simulink model "Simulador_No_lineal"  (R2023a)
settings: Solver=FixedStepAuto  StartTime=0.0  StopTime=70  FixedStep=Ts  RelTol=1e-3
undefined symbols (not defined in the file): IMU1_aB, IMU1_aK, IMU1_aN, IMU1_gB, IMU1_gK, IMU1_gN, IMU2_aB, IMU2_aK, IMU2_aN, IMU2_gB, IMU2_gK, IMU2_gN, IMU3_aB, IMU3_aK, IMU3_aN, IMU3_gB, IMU3_gK, IMU3_gN, Ts, TsMot, TsPos, TsRef, TsSenB, TsSenF, TsVel
libraries: mspsensorlib x3, simulink x1
(part 1 of 3)
settings Model: Creator=rrico  LastModifiedBy=rrico
settings OptimizationCC: ReuseModelBlockBuffer=off

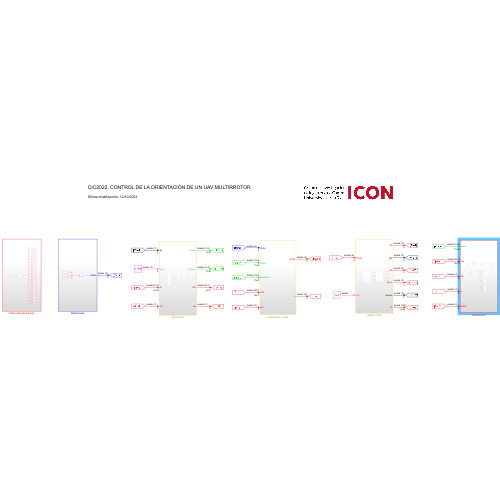
[thumbnail: Simulink's stored preview of the top-level diagram]
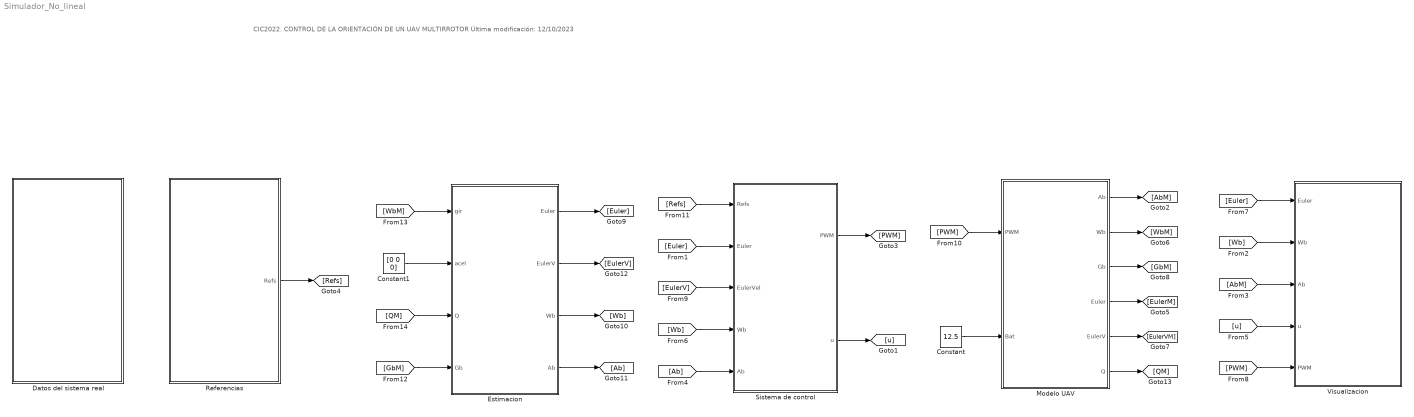
== system Simulador_No_lineal ==
  note: CIC2022. CONTROL DE LA ORIENTACIÓN DE UN UAV MULTIRROTOR
      |
      | Última modificación: 12/10/2023
  Constant : Constant  Value=12.5
  Constant1 : Constant  Value=[0 0 0]
  Datos del sistema real : Subsystem
  Estimacion : Subsystem
  Modelo UAV : Subsystem
  Referencias : Subsystem
  Sistema de control : Subsystem
  Visualizacion : Subsystem
  wires:
  Referencias/1(Refs) -> [Refs]
  [Wb] -> Visualizacion/2(Wb)
  [AbM] -> Visualizacion/3(Ab)
  [PWM] -> Visualizacion/5(PWM)
  [u] -> Visualizacion/4(u)
  Constant/1 -> Modelo UAV/2(Bat)
  Sistema de control/1(PWM) -> [PWM]
  [PWM] -> Modelo UAV/1(PWM)
  Modelo UAV/2(Wb) -> [WbM]
  Modelo UAV/1(Ab) -> [AbM]
  [Refs] -> Sistema de control/1(Refs)
  [Wb] -> Sistema de control/4(Wb)
  Sistema de control/2(u) -> [u]
  [Euler] -> Sistema de control/2(Euler)
  Modelo UAV/4(Euler) -> [EulerM]
  [Euler] -> Visualizacion/1(Euler)
  [Ab] -> Sistema de control/5(Ab)
  Modelo UAV/5(EulerV) -> [EulerVM]
  [EulerV] -> Sistema de control/3(EulerVel)
  Modelo UAV/3(Gb) -> [GbM]
  [WbM] -> Estimacion/1(gir)
  Constant1/1 -> Estimacion/2(acel)
  Estimacion/1(Euler) -> [Euler]
  Estimacion/3(Wb) -> [Wb]
  Estimacion/4(Ab) -> [Ab]
  Estimacion/2(EulerV) -> [EulerV]
  Modelo UAV/6(Q) -> [QM]
  [QM] -> Estimacion/3(Q)
  [GbM] -> Estimacion/4(Gb)

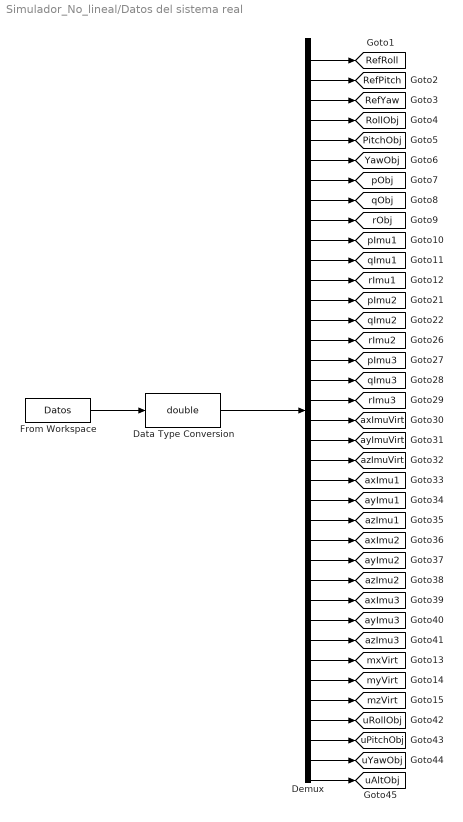
== system Simulador_No_lineal/Datos del sistema real ==
  Data Type Conversion : DataTypeConversion  OutDataTypeStr=double  SaturateOnIntegerOverflow=off  RndMeth=Floor
  Demux : Demux  Outputs=38
  From Workspace : FromWorkspace  VariableName=Datos  SampleTime=Ts
  tag scope: PitchObj=global, RefPitch=global, RefRoll=global, RefYaw=global, RollObj=global, YawObj=global, axImu1=global, axImu2=global, axImu3=global, axImuVirt=global, ayImu1=global, ayImu2=global, ayImu3=global, ayImuVirt=global, azImu1=global, azImu2=global, azImu3=global, azImuVirt=global, mxVirt=global, myVirt=global, mzVirt=global, pImu1=global, pImu2=global, pImu3=global, pObj=global, qImu1=global, qImu2=global, qImu3=global, qObj=global, rImu1=global, rImu2=global, rImu3=global, rObj=global, uAltObj=global, uPitchObj=global, uRollObj=global, uYawObj=global
  wires:
  Demux/31 -> [azImu3]
  Demux/7 -> [YawObj]
  Demux/17 -> [pImu3]
  Demux/25 -> [azImu1]
  Demux/27 -> [ayImu2]
  Demux/16 -> [rImu2]
  Demux/15 -> [qImu2]
  Demux/30 -> [ayImu3]
  Demux/21 -> [ayImuVirt]
  Demux/10 -> [rObj]
  Demux/2 -> [RefRoll]
  Demux/24 -> [ayImu1]
  Demux/5 -> [RollObj]
  Demux/29 -> [axImu3]
  Demux/8 -> [pObj]
  Demux/28 -> [azImu2]
  Demux/18 -> [qImu3]
  Demux/6 -> [PitchObj]
  Demux/19 -> [rImu3]
  Data Type Conversion/1 -> Demux/1
  Demux/4 -> [RefYaw]
  Demux/22 -> [azImuVirt]
  From Workspace/1 -> Data Type Conversion/1
  Demux/23 -> [axImu1]
  Demux/9 -> [qObj]
  Demux/13 -> [rImu1]
  Demux/3 -> [RefPitch]
  Demux/26 -> [axImu2]
  Demux/11 -> [pImu1]
  Demux/14 -> [pImu2]
  Demux/38 -> [uAltObj]
  Demux/37 -> [uYawObj]
  Demux/36 -> [uPitchObj]
  Demux/35 -> [uRollObj]
  Demux/32 -> [mxVirt]
  Demux/33 -> [myVirt]
  Demux/34 -> [mzVirt]
  Demux/20 -> [axImuVirt]
  Demux/12 -> [qImu1]

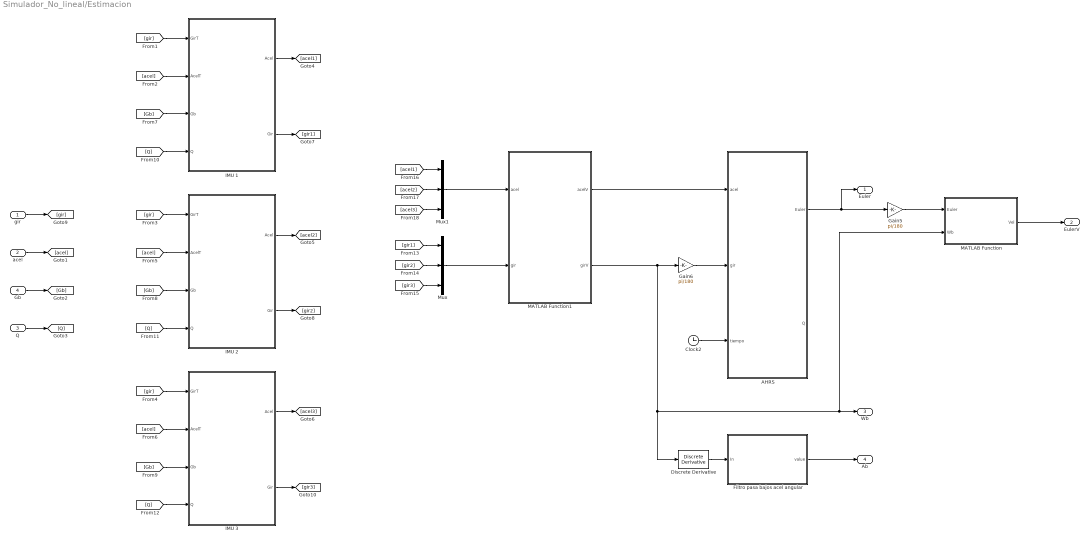
== system Simulador_No_lineal/Estimacion ==
  gir : Inport
  acel : Inport  Port=2
  Q : Inport  Port=3
  Gb : Inport  Port=4
  AHRS : Subsystem  TreatAsAtomicUnit=on  SystemSampleTime=TsPos  mask{T=on, Beta=0.033, Zeta=0.005, Kp=0.5, Ki=0.1}
      mask prompts: T "Filtro Madgwick"
  Clock2 : Clock
  Discrete Derivative : simulink/Discrete/Discrete Derivative  gainval=1.0  ICPrevScaledInput=0.0  OutMin=[]  OutMax=[]  OutDataType=fixdt(1, 16)  OutScaling=2^-10  DoSatur=off
  Filtro pasa bajos acel angular : Subsystem  TreatAsAtomicUnit=on  SystemSampleTime=TsVel  mask{P=2, Fc=30, TsF=TsSenF}
      mask prompts: P "Polos"; Fc "Frecuencia de corte"; TsF "Tiempo de muestreo"
      mask DialogControl ParameterGroup1 Prompt: Parameters
  Gain5 : Gain  Gain=pi/180
  Gain6 : Gain  Gain=pi/180
  IMU 1 : Subsystem  mask{aN=IMU1_aN, aB=IMU1_aB, aK=IMU1_aK, gN=IMU1_gN, gB=IMU1_gB, gK=IMU1_gK, E=on, R=off, ESM=on, EF=on, NP=2, FC=40}
      mask prompts: aN "Velocity random walk"; aB "Bias instability"; aK "Acceleration random walk"; gN "Angle random walk"; gB "Bias instability"; gK "Rate random walk"; E "Activar IMU"; R "Activar ruido externo"; ESM "Activar submuestreo"; EF "Activar filtro"; NP "Numero de polos"; FC "Frecuencia de corte"
      mask DialogControl ParameterGroupVar Prompt: Acelerometro
      mask DialogControl Container3 Prompt: Giroscopio
      mask DialogControl Container4 Prompt: IMU
      mask DialogControl Container5 Prompt: Filtro
  IMU 2 : Subsystem  mask{aN=IMU2_aN, aB=IMU2_aB, aK=IMU2_aK, gN=IMU2_gN, gB=IMU2_gB, gK=IMU2_gK, E=on, R=off, ESM=on, EF=on, NP=2, FC=40}
      mask prompts: aN "Velocity random walk"; aB "Bias instability"; aK "Acceleration random walk"; gN "Angle random walk"; gB "Bias instability"; gK "Rate random walk"; E "Activar IMU"; R "Activar ruido externo"; ESM "Activar submuestreo"; EF "Activar filtro"; NP "Numero de polos"; FC "Frecuencia de corte"
      mask DialogControl ParameterGroupVar Prompt: Acelerometro
      mask DialogControl Container3 Prompt: Giroscopio
      mask DialogControl Container4 Prompt: IMU
      mask DialogControl Container5 Prompt: Filtro
  IMU 3 : Subsystem  mask{aN=IMU3_aN, aB=IMU3_aB, aK=IMU3_aK, gN=IMU3_gN, gB=IMU3_gB, gK=IMU3_gK, E=on, R=off, ESM=on, EF=on, NP=2, FC=40}
      mask prompts: aN "Velocity random walk"; aB "Bias instability"; aK "Acceleration random walk"; gN "Angle random walk"; gB "Bias instability"; gK "Rate random walk"; E "Activar IMU"; R "Activar ruido externo"; ESM "Activar submuestreo"; EF "Activar filtro"; NP "Numero de polos"; FC "Frecuencia de corte"
      mask DialogControl ParameterGroupVar Prompt: Acelerometro
      mask DialogControl Container3 Prompt: Giroscopio
      mask DialogControl Container4 Prompt: IMU
      mask DialogControl Container5 Prompt: Filtro
  MATLAB Function : MATLAB Function  TreatAsAtomicUnit=on  SystemSampleTime=TsPos
  MATLAB Function1 : MATLAB Function  TreatAsAtomicUnit=on  SystemSampleTime=TsSenF
  Mux : Mux  Inputs=3
  Mux1 : Mux  Inputs=3
  Euler : Outport
  EulerV : Outport  Port=2
  Wb : Outport  Port=3
  Ab : Outport  Port=4
  wires:
  Gain6/1 -> AHRS/2(gir)
  AHRS/1(Euler) -> Euler/1, Gain5/1
  Gain5/1 -> MATLAB Function/1(Euler)
  MATLAB Function/1(Vel) -> EulerV/1
  Discrete Derivative/1 -> Filtro pasa bajos acel angular/1(In)
  Filtro pasa bajos acel angular/1(value) -> Ab/1
  Clock2/1 -> AHRS/3(tiempo)
  MATLAB Function1/2(girV) -> Wb/1, MATLAB Function/2(Wb), Discrete Derivative/1, Gain6/1
  gir/1 -> [gir]
  acel/1 -> [acel]
  Gb/1 -> [Gb]
  Q/1 -> [Q]
  [gir] -> IMU 1/1(GirT)
  [gir] -> IMU 2/1(GirT)
  [gir] -> IMU 3/1(GirT)
  [acel] -> IMU 1/2(AcelT)
  [acel] -> IMU 2/2(AcelT)
  [acel] -> IMU 3/2(AcelT)
  [Gb] -> IMU 1/3(Gb)
  [Gb] -> IMU 2/3(Gb)
  [Gb] -> IMU 3/3(Gb)
  [Q] -> IMU 1/4(Q)
  [Q] -> IMU 2/4(Q)
  [Q] -> IMU 3/4(Q)
  IMU 1/1(Acel) -> [acel1]
  IMU 2/1(Acel) -> [acel2]
  IMU 3/1(Acel) -> [acel3]
  IMU 1/2(Gir) -> [gir1]
  IMU 2/2(Gir) -> [gir2]
  IMU 3/2(Gir) -> [gir3]
  [gir1] -> Mux/1
  [gir2] -> Mux/2
  [gir3] -> Mux/3
  [acel1] -> Mux1/1
  [acel2] -> Mux1/2
  [acel3] -> Mux1/3
  Mux1/1 -> MATLAB Function1/1(acel)
  Mux/1 -> MATLAB Function1/2(gir)
  MATLAB Function1/1(acelV) -> AHRS/1(acel)

== system Simulador_No_lineal/Modelo UAV ==
  PWM : Inport
  Bat : Inport  Port=2
  Dinamica UAV : Subsystem  mask{Mo=[0 0 0], B=[0.002 0.005 0.005]*0, F=[0.025 0.006 0.006]*0, I=[0.0014 0.025 0.0549], Im=0.0005, dM=0, M=0.2472, Dr=0.09, Dp=0.0675, Y=off, Mq=on}
      mask prompts: Mo "Par inicial"; B "Rozamiento viscoso"; F "Rozamiento estático"; I "Inercia"; Im "Inercia del rotor"; dM "Distancia del centro de masas"; M "Masa"; Dr "Distancia de los rotores a roll"; Dp "Distancia de los rotores a pitch"; Y "Habilitacion yaw"; Mq "Modelo de maqueta"
      mask DialogControl DescTextVar Prompt: Modelo dinámico del UAV
      mask DialogControl Parameter1 Prompt: Rozamientos y pares adicionales
      mask DialogControl Parameter2 Prompt: Parámetros físicos
      mask DialogControl Parameter3 Prompt: Selectores
  Sistema de propulsion : Subsystem  mask{MF=[-6.7899 14.607 -0.4253 0.0213; -8.4461 16.962 -0.2084 0.0076; -9.5828 18.733 0.1539 -0.0175; -12.165 22.368 -0.0708 -0.018; -12.638 23.102 0.6345 -0.0512], MD=[0.0103 0.0273 0.0082 0.0004; -0.0179 0.0606 0.005 0.0001; 0.0107 0.032 0.0095 0.0002; -0.0117 0.0697 0.0007 0.0007; 0.0227 0.0301 0.0117 -0.0002], MV=[0 -1075.7 3391.3 5.1514; 0 -1117.8 3467.7 31.49; 0 -1464 4031.2 0.4344; 0 -1601.8 4277.8 4.6327; 0 -1710.5 4430.8 10.996], Vmin=12.5, Vmax=16.5, Tau=0.05}
      mask prompts: MF "Matriz de coeficientes fuerza"; MD "Matriz de coeficientes drag"; MV "Matriz de coeficientes velocidad"; Vmin "Voltaje minimo"; Vmax "Voltaje maximo"; Tau "Dinamica"
      mask DialogControl ParameterGroupVar1 Prompt: Estatica del motor
      mask DialogControl ParameterGroupVar2 Prompt: Dinamica del motor
  Ab : Outport
  Wb : Outport  Port=2
  Gb : Outport  Port=3
  Euler : Outport  Port=4
  EulerV : Outport  Port=5
  Q : Outport  Port=6
  wires:
  PWM/1 -> Sistema de propulsion/1(PWM)
  Bat/1 -> Sistema de propulsion/2(v)
  Dinamica UAV/3(Gb) -> Gb/1
  Sistema de propulsion/2(D) -> Dinamica UAV/2(Delta)
  Sistema de propulsion/3(W) -> Dinamica UAV/3(Wm)
  Dinamica UAV/2(Wb) -> Wb/1
  Sistema de propulsion/1(T) -> Dinamica UAV/1(T)
  Dinamica UAV/1(Ab) -> Ab/1
  Dinamica UAV/4(Euler) -> Euler/1
  Dinamica UAV/5(EulerV) -> EulerV/1
  Dinamica UAV/6(Q) -> Q/1

== system Simulador_No_lineal/Referencias ==
  Mux17 : Mux  Inputs=3
  Zero-Order Hold : ZeroOrderHold  SampleTime=TsRef
  Refs : Outport  VectorParamsAs1DForOutWhenUnconnected=off
  wires:
  Zero-Order Hold/1 -> Refs/1
  [RefYaw] -> Mux17/3
  [RefPitch] -> Mux17/2
  [RefRoll] -> Mux17/1
  Mux17/1 -> Zero-Order Hold/1

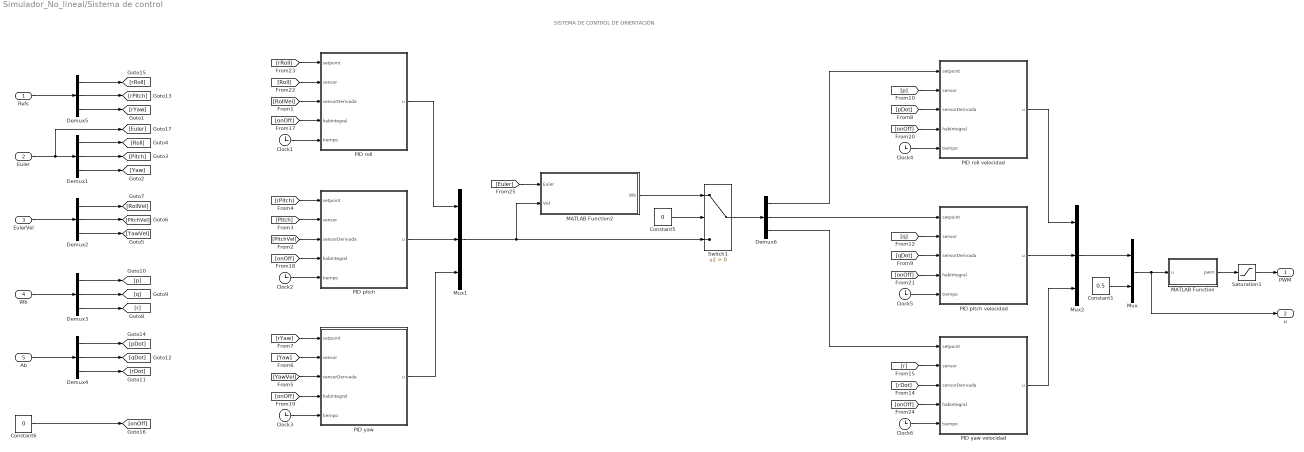
== system Simulador_No_lineal/Sistema de control ==
  note: SISTEMA DE CONTROL DE ORIENTACIÓN
  Refs : Inport
  Euler : Inport  Port=2
  EulerVel : Inport  Port=3
  Wb : Inport  Port=4
  Ab : Inport  Port=5
  Clock{1..6} (6 alike) : Clock
  Constant1 : Constant  Value=0.5  SampleTime=-1
  Constant5 : Constant  Value=0
  Constant6 : Constant  Value=0  SampleTime=-1
  Demux{1..6} (6 alike) : Demux  Outputs=3
  MATLAB Function : MATLAB Function  TreatAsAtomicUnit=on
  MATLAB Function2 : MATLAB Function  TreatAsAtomicUnit=on  SystemSampleTime=TsVel
  Mux : Mux  Inputs=2
  Mux1 : Mux  Inputs=3
  Mux2 : Mux  Inputs=3
  PID pitch : Subsystem  TreatAsAtomicUnit=on  SystemSampleTime=TsPos  mask{Kp=4, Ki=0, Kd=0, Kff=0, LimI=2000, LimT=2000}
      mask prompts: LimI "Limite I"; LimT "Limite total"
  PID pitch velocidad : Subsystem  TreatAsAtomicUnit=on  SystemSampleTime=TsVel  mask{Kp=0.0024, Ki=0.000378, Kd=0, Kff=0, LimI=1, LimT=1}
      mask prompts: LimI "Limite I"; LimT "Limite total"
  PID roll : Subsystem  TreatAsAtomicUnit=on  SystemSampleTime=TsPos  mask{Kp=5, Ki=0, Kd=0, Kff=0, LimI=2000, LimT=2000}
      mask prompts: LimI "Limite I"; LimT "Limite total"
  PID roll velocidad : Subsystem  TreatAsAtomicUnit=on  SystemSampleTime=TsVel  mask{Kp=0.00051, Ki=0.000000153, Kd=0, Kff=0, LimI=1, LimT=1}
      mask prompts: LimI "Limite I"; LimT "Limite total"
  PID yaw : Subsystem  TreatAsAtomicUnit=on  SystemSampleTime=TsPos  mask{Kp=0, Ki=0, Kd=0, Kff=0, LimI=2000, LimT=2000}
      mask prompts: LimI "Limite I"; LimT "Limite total"
  PID yaw velocidad : Subsystem  TreatAsAtomicUnit=on  SystemSampleTime=TsVel  mask{Kp=0, Ki=0, Kd=0, Kff=0, LimI=1, LimT=1}
      mask prompts: LimI "Limite I"; LimT "Limite total"
  Saturation1 : Saturate  UpperLimit=1  LowerLimit=0
  Switch1 : Switch  Criteria=u2 > Threshold  SaturateOnIntegerOverflow=off  InputSameDT=off
  PWM : Outport  VectorParamsAs1DForOutWhenUnconnected=off
  u : Outport  Port=2  VectorParamsAs1DForOutWhenUnconnected=off
  wires:
  Saturation1/1 -> PWM/1
  MATLAB Function/1(pwm) -> Saturation1/1
  Constant1/1 -> Mux/2
  Mux/1 -> u/1, MATLAB Function/1(u)
  [Pitch] -> PID pitch/2(sensor)
  [rPitch] -> PID pitch/1(setpoint)
  [Yaw] -> PID yaw/2(sensor)
  [YawVel] -> PID yaw/3(sensorDerivada)
  [Roll] -> PID roll/2(sensor)
  [RollVel] -> PID roll/3(sensorDerivada)
  [rYaw] -> PID yaw/1(setpoint)
  [rRoll] -> PID roll/1(setpoint)
  PID pitch/1(u) -> Mux1/2
  [onOff] -> PID roll/4(habIntegral)
  PID yaw/1(u) -> Mux1/3
  [PitchVel] -> PID pitch/3(sensorDerivada)
  PID roll/1(u) -> Mux1/1
  PID pitch velocidad/1(u) -> Mux2/2
  PID roll velocidad/1(u) -> Mux2/1
  [p] -> PID roll velocidad/2(sensor)
  Demux6/1 -> PID roll velocidad/1(setpoint)
  [r] -> PID yaw velocidad/2(sensor)
  [pDot] -> PID roll velocidad/3(sensorDerivada)
  Demux6/3 -> PID yaw velocidad/1(setpoint)
  PID yaw velocidad/1(u) -> Mux2/3
  Demux6/2 -> PID pitch velocidad/1(setpoint)
  [qDot] -> PID pitch velocidad/3(sensorDerivada)
  Mux2/1 -> Mux/1
  [q] -> PID pitch velocidad/2(sensor)
  [rDot] -> PID yaw velocidad/3(sensorDerivada)
  Demux1/2 -> [Pitch]
  Demux2/1 -> [RollVel]
  Demux5/1 -> [rRoll]
  Demux5/3 -> [rYaw]
  Demux2/3 -> [YawVel]
  Demux1/3 -> [Yaw]
  Demux1/1 -> [Roll]
  Demux2/2 -> [PitchVel]
  Demux5/2 -> [rPitch]
  Demux3/2 -> [q]
  Demux3/1 -> [p]
  Demux4/3 -> [rDot]
  Demux3/3 -> [r]
  Demux4/1 -> [pDot]
  Demux4/2 -> [qDot]
  Constant6/1 -> [onOff]
  [onOff] -> PID pitch/4(habIntegral)
  Clock1/1 -> PID roll/5(tiempo)
  [onOff] -> PID yaw/4(habIntegral)
  [onOff] -> PID roll velocidad/4(habIntegral)
  [onOff] -> PID pitch velocidad/4(habIntegral)
  [onOff] -> PID yaw velocidad/4(habIntegral)
  Constant5/1 -> Switch1/2
  MATLAB Function2/1(Wb) -> Switch1/1
  Mux1/1 -> MATLAB Function2/2(Vel), Switch1/3
  [Euler] -> MATLAB Function2/1(Euler)
  Switch1/1 -> Demux6/1
  Ab/1 -> Demux4/1
  Wb/1 -> Demux3/1
  EulerVel/1 -> Demux2/1
  Euler/1 -> [Euler], Demux1/1
  Refs/1 -> Demux5/1
  Clock2/1 -> PID pitch/5(tiempo)
  Clock3/1 -> PID yaw/5(tiempo)
  Clock4/1 -> PID roll velocidad/5(tiempo)
  Clock5/1 -> PID pitch velocidad/5(tiempo)
  Clock6/1 -> PID yaw velocidad/5(tiempo)

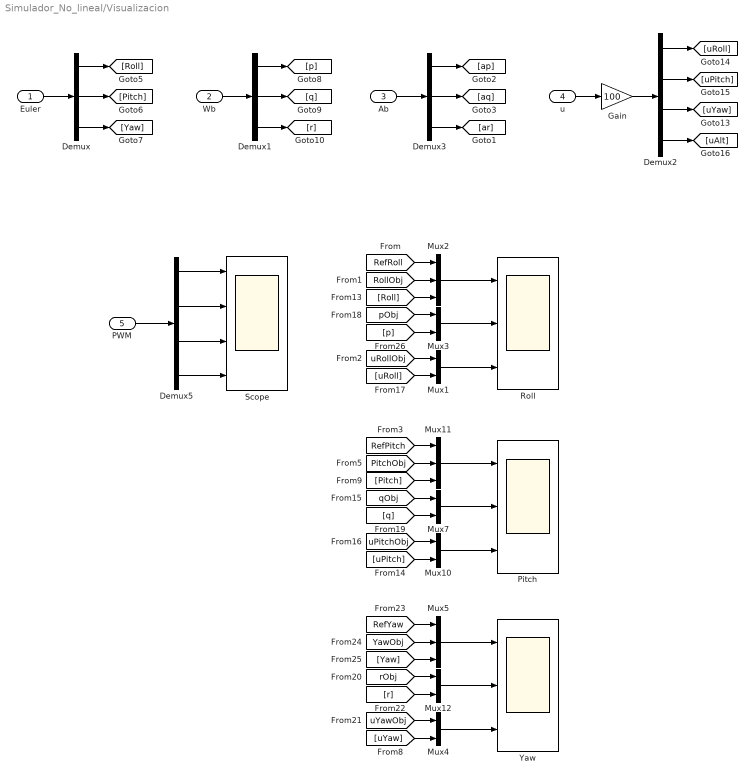
== system Simulador_No_lineal/Visualizacion ==
  Euler : Inport
  Wb : Inport  Port=2
  Ab : Inport  Port=3
  u : Inport  Port=4
  PWM : Inport  Port=5
  Demux : Demux  Outputs=3
  Demux1 : Demux  Outputs=3
  Demux2 : Demux
  Demux3 : Demux  Outputs=3
  Demux5 : Demux
  Gain : Gain  Gain=100
  Mux{1,3..4,7,10,12} (6 alike) : Mux  Inputs=2
  Mux11 : Mux  Inputs=3
  Mux2 : Mux  Inputs=3
  Mux5 : Mux  Inputs=3
  Pitch : Scope  NumInputPorts=3
  Roll : Scope  NumInputPorts=3
  Scope : Scope  NumInputPorts=4
  Yaw : Scope  NumInputPorts=3
  wires:
  [YawObj] -> Mux5/2
  [r] -> Mux12/2
  Mux11/1 -> Pitch/1
  [uYawObj] -> Mux4/1
  Demux/3 -> [Yaw]
  [uPitchObj] -> Mux10/1
  [RefYaw] -> Mux5/1
  Demux1/2 -> [q]
  Euler/1 -> Demux/1
  [Yaw] -> Mux5/3
  Demux/2 -> [Pitch]
  [rObj] -> Mux12/1
  Demux1/1 -> [p]
  [q] -> Mux7/2
  Wb/1 -> Demux1/1
  Demux1/3 -> [r]
  [qObj] -> Mux7/1
  Demux/1 -> [Roll]
  [uYaw] -> Mux4/2
  Demux2/3 -> [uYaw]
  Demux2/2 -> [uPitch]
  Demux2/1 -> [uRoll]
  u/1 -> Gain/1
  [PitchObj] -> Mux11/2
  [RefPitch] -> Mux11/1
  [Pitch] -> Mux11/3
  Demux2/4 -> [uAlt]
  Mux10/1 -> Pitch/3
  Mux7/1 -> Pitch/2
  [uPitch] -> Mux10/2
  Mux5/1 -> Yaw/1
  Mux12/1 -> Yaw/2
  Mux4/1 -> Yaw/3
  Demux3/3 -> [ar]
  Ab/1 -> Demux3/1
  Demux3/1 -> [ap]
  Demux3/2 -> [aq]
  Gain/1 -> Demux2/1
  PWM/1 -> Demux5/1
  Demux5/1 -> Scope/1
  Demux5/3 -> Scope/3
  Demux5/2 -> Scope/2
  Demux5/4 -> Scope/4
  [uRoll] -> Mux1/2
  [Roll] -> Mux2/3
  Mux2/1 -> Roll/1
  Mux1/1 -> Roll/3
  [RollObj] -> Mux2/2
  [pObj] -> Mux3/1
  [p] -> Mux3/2
  Mux3/1 -> Roll/2
  [RefRoll] -> Mux2/1
  [uRollObj] -> Mux1/1

== system Simulador_No_lineal/Estimacion/AHRS ==
  acel : Inport
  gir : Inport  Port=2
  tiempo : Inport  Port=3
  Constant1 : Constant  Value=T
  Constant2 : Constant  Value=Beta
  Constant3 : Constant  Value=Zeta
  Constant4 : Constant  Value=Ki
  Constant5 : Constant  Value=Kp
  Gain : Gain  Gain=2
  Gain1 : Gain  Gain=2
  Gain2 : Gain  Gain=2
  MATLAB Function : MATLAB Function
  MATLAB Function2 : MATLAB Function
  MATLAB Function4 : MATLAB Function
  Switch : Switch  Criteria=u2 > Threshold  SaturateOnIntegerOverflow=off  InputSameDT=off
  Euler : Outport
  Q : Outport  Port=2
  wires:
  Constant1/1 -> Switch/2
  gir/1 -> MATLAB Function/3(gir), MATLAB Function2/3(gir)
  Constant5/1 -> Gain1/1
  MATLAB Function/1(Q) -> Switch/1
  Constant2/1 -> Gain/1
  Constant3/1 -> MATLAB Function/1(zeta)
  Constant4/1 -> Gain2/1
  MATLAB Function2/1(Q) -> Switch/3
  tiempo/1 -> MATLAB Function/5(tiempo), MATLAB Function2/5(tiempo)
  acel/1 -> MATLAB Function/4(acel), MATLAB Function2/4(acel)
  Gain/1 -> MATLAB Function/2(beta)
  Gain1/1 -> MATLAB Function2/1(kp)
  Gain2/1 -> MATLAB Function2/2(ki)
  Switch/1 -> MATLAB Function4/1(Q), Q/1
  MATLAB Function4/1(Euler) -> Euler/1

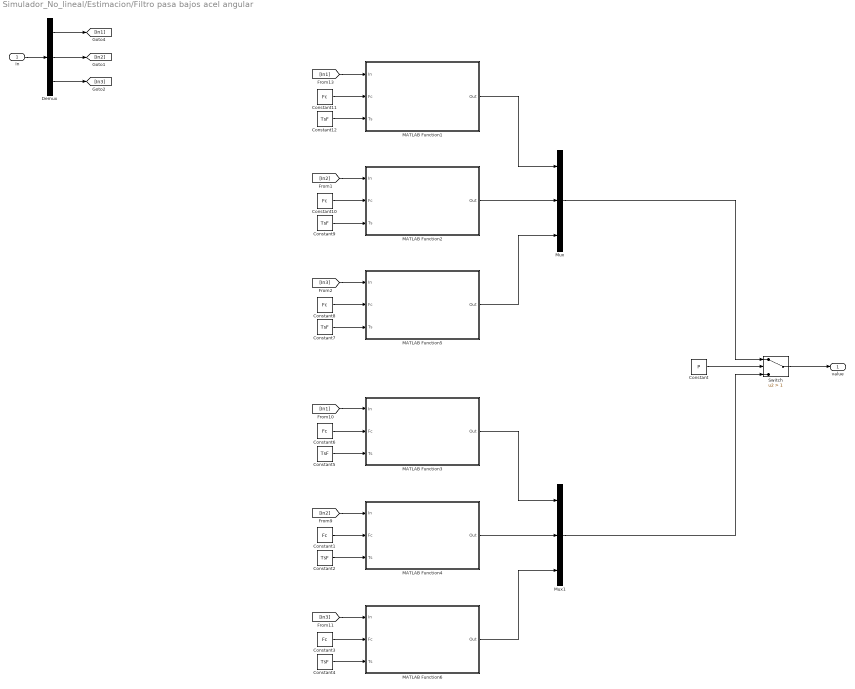
== system Simulador_No_lineal/Estimacion/Filtro pasa bajos acel angular ==
  In : Inport
  Constant : Constant  Value=P
  Constant{1,3,6,8,10..11} (6 alike) : Constant  Value=Fc
  Constant{2,4..5,7,9,12} (6 alike) : Constant  Value=TsF
  Demux : Demux  Outputs=3
  MATLAB Function1 : MATLAB Function  TreatAsAtomicUnit=on
  MATLAB Function2 : MATLAB Function  TreatAsAtomicUnit=on
  MATLAB Function3 : MATLAB Function  TreatAsAtomicUnit=on
  MATLAB Function4 : MATLAB Function  TreatAsAtomicUnit=on
  MATLAB Function5 : MATLAB Function  TreatAsAtomicUnit=on
  MATLAB Function6 : MATLAB Function  TreatAsAtomicUnit=on
  Mux : Mux  Inputs=3
  Mux1 : Mux  Inputs=3
  Switch : Switch  Criteria=u2 > Threshold  Threshold=1  SaturateOnIntegerOverflow=off  InputSameDT=off
  value : Outport
  wires:
  Constant/1 -> Switch/2
  Switch/1 -> value/1
  [In1] -> MATLAB Function1/1(In)
  MATLAB Function2/1(Out) -> Mux/2
  MATLAB Function1/1(Out) -> Mux/1
  MATLAB Function5/1(Out) -> Mux/3
  Mux/1 -> Switch/1
  In/1 -> Demux/1
  Demux/1 -> [In1]
  Demux/2 -> [In2]
  Demux/3 -> [In3]
  [In2] -> MATLAB Function2/1(In)
  [In3] -> MATLAB Function5/1(In)
  Constant4/1 -> MATLAB Function6/3(Ts)
  Constant3/1 -> MATLAB Function6/2(Fc)
  Constant1/1 -> MATLAB Function4/2(Fc)
  Constant2/1 -> MATLAB Function4/3(Ts)
  [In3] -> MATLAB Function6/1(In)
  [In2] -> MATLAB Function4/1(In)
  [In1] -> MATLAB Function3/1(In)
  MATLAB Function3/1(Out) -> Mux1/1
  MATLAB Function4/1(Out) -> Mux1/2
  MATLAB Function6/1(Out) -> Mux1/3
  Mux1/1 -> Switch/3
  Constant5/1 -> MATLAB Function3/3(Ts)
  Constant6/1 -> MATLAB Function3/2(Fc)
  Constant7/1 -> MATLAB Function5/3(Ts)
  Constant8/1 -> MATLAB Function5/2(Fc)
  Constant10/1 -> MATLAB Function2/2(Fc)
  Constant9/1 -> MATLAB Function2/3(Ts)
  Constant12/1 -> MATLAB Function1/3(Ts)
  Constant11/1 -> MATLAB Function1/2(Fc)

== system Simulador_No_lineal/Estimacion/IMU 1 ==
  note: cnt
  GirT : Inport
  AcelT : Inport  Port=2
  Gb : Inport  Port=3
  Q : Inport  Port=4
  Constant : Constant  Value=ESM
  Constant1 : Constant  Value=20
  Constant2 : Constant  Value=20
  Constant3 : Constant  Value=ESM
  Constant4 : Constant  Value=EF
  Constant5 : Constant  Value=E
  Constant6 : Constant  Value=EF
  Constant7 : Constant  Value=E
  Data Store Memory : DataStoreMemory  DataStoreName=acumW1  WriteAfterWriteMsg=warning  InitialValue=[0 0 0]  ShowAdditionalParam=off  OutDataTypeStr=double  Dimensions=3
  Data Store Memory1 : DataStoreMemory  DataStoreName=cntW1  WriteAfterWriteMsg=warning  ShowAdditionalParam=off  OutDataTypeStr=double
  Data Store Memory2 : DataStoreMemory  DataStoreName=acumA1  WriteAfterWriteMsg=warning  InitialValue=[0 0 0]  ShowAdditionalParam=off  OutDataTypeStr=double  Dimensions=3
  Data Store Memory3 : DataStoreMemory  DataStoreName=cntA1  WriteAfterWriteMsg=warning  ShowAdditionalParam=off  OutDataTypeStr=double
  Filtro pasa bajos  acelerometro : Subsystem  TreatAsAtomicUnit=on  SystemSampleTime=TsSenF  mask{P=NP, Fc=FC, TsF=TsSenF}
      mask prompts: P "Polos"; Fc "Frecuencia de corte"; TsF "Tiempo de muestreo"
      mask DialogControl ParameterGroup1 Prompt: Parameters
  Filtro pasa bajos giroscopio : Subsystem  TreatAsAtomicUnit=on  SystemSampleTime=TsSenF  mask{P=NP, Fc=FC, TsF=TsSenF}
      mask prompts: P "Polos"; Fc "Frecuencia de corte"; TsF "Tiempo de muestreo"
      mask DialogControl ParameterGroup1 Prompt: Parameters
  MATLAB Function1 : MATLAB Function  TreatAsAtomicUnit=on  SystemSampleTime=TsSenB
  MATLAB Function2 : MATLAB Function  TreatAsAtomicUnit=on  SystemSampleTime=TsSenF
  MATLAB Function3 : MATLAB Function  TreatAsAtomicUnit=on  SystemSampleTime=TsSenF
  MATLAB Function4 : MATLAB Function  TreatAsAtomicUnit=on  SystemSampleTime=TsSenB
  Sensor IMU : Subsystem
  Switch{1..6} (6 alike) : Switch  Criteria=u2 > Threshold  SaturateOnIntegerOverflow=off  InputSameDT=off
  Acel : Outport
  Gir : Outport  Port=2
  wires:
  Constant4/1 -> Switch3/2
  MATLAB Function3/1(y) -> Switch1/1
  Filtro pasa bajos giroscopio/1(value) -> Switch4/1
  Switch2/1 -> Switch4/3, Filtro pasa bajos giroscopio/1(In)
  Gb/1 -> Switch5/3
  Constant/1 -> Switch2/2
  Switch3/1 -> Acel/1
  Switch5/1 -> Switch1/3, MATLAB Function4/1(u)
  GirT/1 -> Sensor IMU/1(GirT), [gir]
  Filtro pasa bajos  acelerometro/1(value) -> Switch3/1
  Constant3/1 -> Switch1/2
  [gir] -> Switch6/3
  Constant5/1 -> Switch6/2
  Constant2/1 -> MATLAB Function4/2(max)
  Constant6/1 -> Switch4/2
  Switch6/1 -> MATLAB Function1/1(u), Switch2/3
  Sensor IMU/1(AcelB) -> Switch5/1
  Switch1/1 -> Filtro pasa bajos  acelerometro/1(In), Switch3/3
  Constant7/1 -> Switch5/2
  Switch4/1 -> Gir/1
  MATLAB Function2/1(y) -> Switch2/1
  Sensor IMU/2(VelB) -> Switch6/1
  Constant1/1 -> MATLAB Function1/2(max)
  Q/1 -> Sensor IMU/3(Q)
  AcelT/1 -> Sensor IMU/2(AcelT)

== system Simulador_No_lineal/Estimacion/IMU 2 ==
  note: cnt
  GirT : Inport
  AcelT : Inport  Port=2
  Gb : Inport  Port=3
  Q : Inport  Port=4
  Constant : Constant  Value=ESM
  Constant1 : Constant  Value=20
  Constant2 : Constant  Value=20
  Constant3 : Constant  Value=ESM
  Constant4 : Constant  Value=EF
  Constant5 : Constant  Value=E
  Constant6 : Constant  Value=EF
  Constant7 : Constant  Value=E
  Data Store Memory : DataStoreMemory  DataStoreName=acumW2  WriteAfterWriteMsg=warning  InitialValue=[0 0 0]  ShowAdditionalParam=off  OutDataTypeStr=double  Dimensions=3
  Data Store Memory1 : DataStoreMemory  DataStoreName=cntW2  WriteAfterWriteMsg=warning  ShowAdditionalParam=off  OutDataTypeStr=double
  Data Store Memory2 : DataStoreMemory  DataStoreName=acumA2  WriteAfterWriteMsg=warning  InitialValue=[0 0 0]  ShowAdditionalParam=off  OutDataTypeStr=double  Dimensions=3
  Data Store Memory3 : DataStoreMemory  DataStoreName=cntA2  WriteAfterWriteMsg=warning  ShowAdditionalParam=off  OutDataTypeStr=double
  Filtro pasa bajos  acelerometro : Subsystem  TreatAsAtomicUnit=on  SystemSampleTime=TsSenF  mask{P=NP, Fc=FC, TsF=TsSenF}
      mask prompts: P "Polos"; Fc "Frecuencia de corte"; TsF "Tiempo de muestreo"
      mask DialogControl ParameterGroup1 Prompt: Parameters
  Filtro pasa bajos giroscopio : Subsystem  TreatAsAtomicUnit=on  SystemSampleTime=TsSenF  mask{P=NP, Fc=FC, TsF=TsSenF}
      mask prompts: P "Polos"; Fc "Frecuencia de corte"; TsF "Tiempo de muestreo"
      mask DialogControl ParameterGroup1 Prompt: Parameters
  MATLAB Function1 : MATLAB Function  TreatAsAtomicUnit=on  SystemSampleTime=TsSenB
  MATLAB Function2 : MATLAB Function  TreatAsAtomicUnit=on  SystemSampleTime=TsSenF
  MATLAB Function3 : MATLAB Function  TreatAsAtomicUnit=on  SystemSampleTime=TsSenF
  MATLAB Function4 : MATLAB Function  TreatAsAtomicUnit=on  SystemSampleTime=TsSenB
  Sensor IMU : Subsystem
  Switch{1..6} (6 alike) : Switch  Criteria=u2 > Threshold  SaturateOnIntegerOverflow=off  InputSameDT=off
  Acel : Outport
  Gir : Outport  Port=2
  wires:
  AcelT/1 -> Sensor IMU/2(AcelT)
  Q/1 -> Sensor IMU/3(Q)
  Constant1/1 -> MATLAB Function1/2(max)
  Sensor IMU/2(VelB) -> Switch6/1
  MATLAB Function2/1(y) -> Switch2/1
  Switch4/1 -> Gir/1
  Constant7/1 -> Switch5/2
  Switch1/1 -> Switch3/3, Filtro pasa bajos  acelerometro/1(In)
  Sensor IMU/1(AcelB) -> Switch5/1
  Switch6/1 -> Switch2/3, MATLAB Function1/1(u)
  Constant6/1 -> Switch4/2
  Constant2/1 -> MATLAB Function4/2(max)
  Constant5/1 -> Switch6/2
  [gir] -> Switch6/3
  Constant3/1 -> Switch1/2
  Filtro pasa bajos  acelerometro/1(value) -> Switch3/1
  GirT/1 -> [gir], Sensor IMU/1(GirT)
  Switch5/1 -> MATLAB Function4/1(u), Switch1/3
  Switch3/1 -> Acel/1
  Constant/1 -> Switch2/2
  Gb/1 -> Switch5/3
  Switch2/1 -> Filtro pasa bajos giroscopio/1(In), Switch4/3
  Filtro pasa bajos giroscopio/1(value) -> Switch4/1
  MATLAB Function3/1(y) -> Switch1/1
  Constant4/1 -> Switch3/2

== system Simulador_No_lineal/Estimacion/IMU 3 ==
  note: cnt
  GirT : Inport
  AcelT : Inport  Port=2
  Gb : Inport  Port=3
  Q : Inport  Port=4
  Constant : Constant  Value=ESM
  Constant1 : Constant  Value=20
  Constant2 : Constant  Value=20
  Constant3 : Constant  Value=ESM
  Constant4 : Constant  Value=EF
  Constant5 : Constant  Value=E
  Constant6 : Constant  Value=EF
  Constant7 : Constant  Value=E
  Data Store Memory : DataStoreMemory  DataStoreName=acumW3  WriteAfterWriteMsg=warning  InitialValue=[0 0 0]  ShowAdditionalParam=off  OutDataTypeStr=double  Dimensions=3
  Data Store Memory1 : DataStoreMemory  DataStoreName=cntW3  WriteAfterWriteMsg=warning  ShowAdditionalParam=off  OutDataTypeStr=double
  Data Store Memory2 : DataStoreMemory  DataStoreName=acumA3  WriteAfterWriteMsg=warning  InitialValue=[0 0 0]  ShowAdditionalParam=off  OutDataTypeStr=double  Dimensions=3
  Data Store Memory3 : DataStoreMemory  DataStoreName=cntA3  WriteAfterWriteMsg=warning  ShowAdditionalParam=off  OutDataTypeStr=double
  Filtro pasa bajos  acelerometro : Subsystem  TreatAsAtomicUnit=on  SystemSampleTime=TsSenF  mask{P=NP, Fc=FC, TsF=TsSenF}
      mask prompts: P "Polos"; Fc "Frecuencia de corte"; TsF "Tiempo de muestreo"
      mask DialogControl ParameterGroup1 Prompt: Parameters
  Filtro pasa bajos giroscopio : Subsystem  TreatAsAtomicUnit=on  SystemSampleTime=TsSenF  mask{P=NP, Fc=FC, TsF=TsSenF}
      mask prompts: P "Polos"; Fc "Frecuencia de corte"; TsF "Tiempo de muestreo"
      mask DialogControl ParameterGroup1 Prompt: Parameters
  MATLAB Function1 : MATLAB Function  TreatAsAtomicUnit=on  SystemSampleTime=TsSenB
  MATLAB Function2 : MATLAB Function  TreatAsAtomicUnit=on  SystemSampleTime=TsSenF
  MATLAB Function3 : MATLAB Function  TreatAsAtomicUnit=on  SystemSampleTime=TsSenF
  MATLAB Function4 : MATLAB Function  TreatAsAtomicUnit=on  SystemSampleTime=TsSenB
  Sensor IMU : Subsystem
  Switch{1..6} (6 alike) : Switch  Criteria=u2 > Threshold  SaturateOnIntegerOverflow=off  InputSameDT=off
  Acel : Outport
  Gir : Outport  Port=2
  wires:
  Constant4/1 -> Switch3/2
  MATLAB Function3/1(y) -> Switch1/1
  Filtro pasa bajos giroscopio/1(value) -> Switch4/1
  Switch2/1 -> Switch4/3, Filtro pasa bajos giroscopio/1(In)
  Gb/1 -> Switch5/3
  Constant/1 -> Switch2/2
  Switch3/1 -> Acel/1
  Switch5/1 -> Switch1/3, MATLAB Function4/1(u)
  GirT/1 -> Sensor IMU/1(GirT), [gir]
  Filtro pasa bajos  acelerometro/1(value) -> Switch3/1
  Constant3/1 -> Switch1/2
  [gir] -> Switch6/3
  Constant5/1 -> Switch6/2
  Constant2/1 -> MATLAB Function4/2(max)
  Constant6/1 -> Switch4/2
  Switch6/1 -> MATLAB Function1/1(u), Switch2/3
  Sensor IMU/1(AcelB) -> Switch5/1
  Switch1/1 -> Filtro pasa bajos  acelerometro/1(In), Switch3/3
  Constant7/1 -> Switch5/2
  Switch4/1 -> Gir/1
  MATLAB Function2/1(y) -> Switch2/1
  Sensor IMU/2(VelB) -> Switch6/1
  Constant1/1 -> MATLAB Function1/2(max)
  Q/1 -> Sensor IMU/3(Q)
  AcelT/1 -> Sensor IMU/2(AcelT)

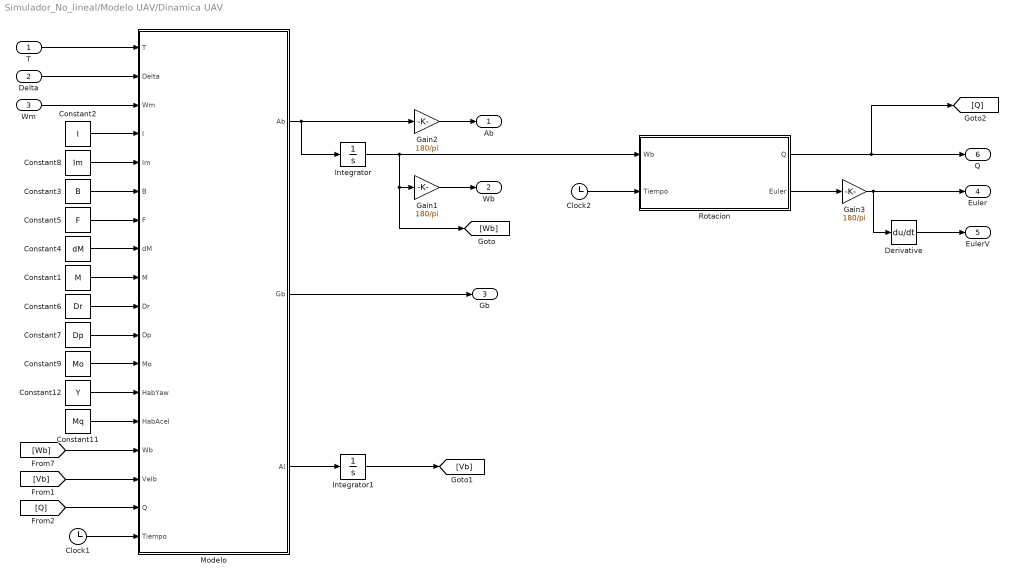
== system Simulador_No_lineal/Modelo UAV/Dinamica UAV ==
  T : Inport
  Delta : Inport  Port=2
  Wm : Inport  Port=3
  Clock1 : Clock
  Clock2 : Clock
  Constant1 : Constant  Value=M
  Constant11 : Constant  Value=Mq
  Constant12 : Constant  Value=Y
  Constant2 : Constant  Value=I
  Constant3 : Constant  Value=B
  Constant4 : Constant  Value=dM
  Constant5 : Constant  Value=F
  Constant6 : Constant  Value=Dr
  Constant7 : Constant  Value=Dp
  Constant8 : Constant  Value=Im
  Constant9 : Constant  Value=Mo
  Derivative : Derivative
  Gain1 : Gain  Gain=180/pi
  Gain2 : Gain  Gain=180/pi
  Gain3 : Gain  Gain=180/pi
  Integrator : Integrator
  Integrator1 : Integrator
  Modelo : MATLAB Function
  Rotacion : MATLAB Function
  Ab : Outport  VectorParamsAs1DForOutWhenUnconnected=off
  Wb : Outport  Port=2  VectorParamsAs1DForOutWhenUnconnected=off
  Gb : Outport  Port=3  VectorParamsAs1DForOutWhenUnconnected=off
  Euler : Outport  Port=4  VectorParamsAs1DForOutWhenUnconnected=off
  EulerV : Outport  Port=5  VectorParamsAs1DForOutWhenUnconnected=off
  Q : Outport  Port=6  VectorParamsAs1DForOutWhenUnconnected=off
  wires:
  Wm/1 -> Modelo/3(Wm)
  Delta/1 -> Modelo/2(Delta)
  T/1 -> Modelo/1(T)
  Constant4/1 -> Modelo/8(dM)
  Constant6/1 -> Modelo/10(Dr)
  Constant8/1 -> Modelo/5(Im)
  Constant3/1 -> Modelo/6(B)
  Constant1/1 -> Modelo/9(M)
  Constant9/1 -> Modelo/12(Mo)
  Modelo/2(Gb) -> Gb/1
  Constant2/1 -> Modelo/4(I)
  Constant5/1 -> Modelo/7(F)
  Integrator/1 -> Gain1/1, [Wb], Rotacion/1(Wb)
  Modelo/1(Ab) -> Integrator/1, Gain2/1
  Constant7/1 -> Modelo/11(Dp)
  Gain1/1 -> Wb/1
  Gain2/1 -> Ab/1
  Constant12/1 -> Modelo/13(HabYaw)
  Clock2/1 -> Rotacion/2(Tiempo)
  [Wb] -> Modelo/15(Wb)
  Gain3/1 -> Euler/1, Derivative/1
  Derivative/1 -> EulerV/1
  Clock1/1 -> Modelo/18(Tiempo)
  Integrator1/1 -> [Vb]
  [Vb] -> Modelo/16(Velb)
  Rotacion/1(Q) -> Q/1, [Q]
  [Q] -> Modelo/17(Q)
  Rotacion/2(Euler) -> Gain3/1
  Constant11/1 -> Modelo/14(HabAcel)
  Modelo/3(Al) -> Integrator1/1

== system Simulador_No_lineal/Modelo UAV/Sistema de propulsion ==
  PWM : Inport
  v : Inport  Port=2
  Constant : Constant  Value=Vmin
  Constant1 : Constant  Value=MF
  Constant2 : Constant  Value=Vmax
  Constant3 : Constant  Value=Vmin
  Constant4 : Constant  Value=MF
  Constant5 : Constant  Value=Vmax
  Constant6 : Constant  Value=Vmin
  Constant7 : Constant  Value=MF
  Constant8 : Constant  Value=Vmax
  Demux : Demux
  MATLAB Function1 : MATLAB Function  TreatAsAtomicUnit=on
  MATLAB Function2 : MATLAB Function  TreatAsAtomicUnit=on
  MATLAB Function3 : MATLAB Function  TreatAsAtomicUnit=on
  Mux : Mux
  Transfer Fcn{1..4} (4 alike) : TransferFcn  Denominator=[Tau 1]
  Zero-Order Hold : ZeroOrderHold  SampleTime=TsMot
  T : Outport
  D : Outport  Port=2
  W : Outport  Port=3
  wires:
  Constant/1 -> MATLAB Function2/3(vMin)
  MATLAB Function2/1(y) -> T/1
  Constant1/1 -> MATLAB Function2/5(m)
  MATLAB Function1/1(y) -> D/1
  v/1 -> MATLAB Function3/2(v), MATLAB Function1/2(v), MATLAB Function2/2(v)
  MATLAB Function3/1(y) -> W/1
  Mux/1 -> MATLAB Function3/1(u), MATLAB Function1/1(u), MATLAB Function2/1(u)
  Constant2/1 -> MATLAB Function2/4(vMax)
  Constant5/1 -> MATLAB Function1/4(vMax)
  Constant4/1 -> MATLAB Function1/5(m)
  Constant3/1 -> MATLAB Function1/3(vMin)
  Constant6/1 -> MATLAB Function3/3(vMin)
  Constant7/1 -> MATLAB Function3/5(m)
  Constant8/1 -> MATLAB Function3/4(vMax)
  Transfer Fcn3/1 -> Mux/1
  Demux/2 -> Transfer Fcn2/1
  Transfer Fcn2/1 -> Mux/2
  Transfer Fcn1/1 -> Mux/3
  Demux/3 -> Transfer Fcn1/1
  Demux/1 -> Transfer Fcn3/1
  Transfer Fcn4/1 -> Mux/4
  Demux/4 -> Transfer Fcn4/1
  Zero-Order Hold/1 -> Demux/1
  PWM/1 -> Zero-Order Hold/1

== system Simulador_No_lineal/Sistema de control/PID pitch ==
  setpoint : Inport
  sensor : Inport  Port=2
  sensorDerivada : Inport  Port=3
  habIntegral : Inport  Port=4
  tiempo : Inport  Port=5
  Constant : Constant  Value=Kp
  Constant1 : Constant  Value=Ki
  Constant2 : Constant  Value=Kd
  Constant3 : Constant  Value=Kff
  Constant4 : Constant  Value=LimI
  Constant5 : Constant  Value=LimT
  MATLAB Function : MATLAB Function  TreatAsAtomicUnit=on
  u : Outport
  wires:
  MATLAB Function/1(u) -> u/1
  tiempo/1 -> MATLAB Function/11(tiempo)
  sensor/1 -> MATLAB Function/8(sensor)
  setpoint/1 -> MATLAB Function/7(setPoint)
  sensorDerivada/1 -> MATLAB Function/9(sensorDerivada)
  Constant1/1 -> MATLAB Function/2(ki)
  Constant3/1 -> MATLAB Function/4(kff)
  Constant4/1 -> MATLAB Function/5(limIntegral)
  Constant5/1 -> MATLAB Function/6(limTotal)
  habIntegral/1 -> MATLAB Function/10(habIntegral)
  Constant2/1 -> MATLAB Function/3(kd)
  Constant/1 -> MATLAB Function/1(kp)

== system Simulador_No_lineal/Sistema de control/PID pitch velocidad ==
  setpoint : Inport
  sensor : Inport  Port=2
  sensorDerivada : Inport  Port=3
  habIntegral : Inport  Port=4
  tiempo : Inport  Port=5
  Constant : Constant  Value=Kp
  Constant1 : Constant  Value=Ki
  Constant2 : Constant  Value=Kd
  Constant3 : Constant  Value=Kff
  Constant4 : Constant  Value=LimI
  Constant5 : Constant  Value=LimT
  MATLAB Function : MATLAB Function  TreatAsAtomicUnit=on
  u : Outport
  wires:
  Constant/1 -> MATLAB Function/1(kp)
  Constant2/1 -> MATLAB Function/3(kd)
  habIntegral/1 -> MATLAB Function/10(habIntegral)
  Constant5/1 -> MATLAB Function/6(limTotal)
  Constant4/1 -> MATLAB Function/5(limIntegral)
  Constant3/1 -> MATLAB Function/4(kff)
  Constant1/1 -> MATLAB Function/2(ki)
  sensorDerivada/1 -> MATLAB Function/9(sensorDerivada)
  setpoint/1 -> MATLAB Function/7(setPoint)
  sensor/1 -> MATLAB Function/8(sensor)
  tiempo/1 -> MATLAB Function/11(tiempo)
  MATLAB Function/1(u) -> u/1

== system Simulador_No_lineal/Sistema de control/PID roll ==
  setpoint : Inport
  sensor : Inport  Port=2
  sensorDerivada : Inport  Port=3
  habIntegral : Inport  Port=4
  tiempo : Inport  Port=5
  Constant : Constant  Value=Kp
  Constant1 : Constant  Value=Ki
  Constant2 : Constant  Value=Kd
  Constant3 : Constant  Value=Kff
  Constant4 : Constant  Value=LimI
  Constant5 : Constant  Value=LimT
  MATLAB Function : MATLAB Function  TreatAsAtomicUnit=on
  u : Outport
  wires:
  Constant/1 -> MATLAB Function/1(kp)
  Constant2/1 -> MATLAB Function/3(kd)
  habIntegral/1 -> MATLAB Function/10(habIntegral)
  Constant5/1 -> MATLAB Function/6(limTotal)
  Constant4/1 -> MATLAB Function/5(limIntegral)
  Constant3/1 -> MATLAB Function/4(kff)
  Constant1/1 -> MATLAB Function/2(ki)
  sensorDerivada/1 -> MATLAB Function/9(sensorDerivada)
  setpoint/1 -> MATLAB Function/7(setPoint)
  sensor/1 -> MATLAB Function/8(sensor)
  tiempo/1 -> MATLAB Function/11(tiempo)
  MATLAB Function/1(u) -> u/1

== system Simulador_No_lineal/Sistema de control/PID roll velocidad ==
  setpoint : Inport
  sensor : Inport  Port=2
  sensorDerivada : Inport  Port=3
  habIntegral : Inport  Port=4
  tiempo : Inport  Port=5
  Constant : Constant  Value=Kp
  Constant1 : Constant  Value=Ki
  Constant2 : Constant  Value=Kd
  Constant3 : Constant  Value=Kff
  Constant4 : Constant  Value=LimI
  Constant5 : Constant  Value=LimT
  MATLAB Function : MATLAB Function  TreatAsAtomicUnit=on
  u : Outport
  wires:
  MATLAB Function/1(u) -> u/1
  tiempo/1 -> MATLAB Function/11(tiempo)
  sensor/1 -> MATLAB Function/8(sensor)
  setpoint/1 -> MATLAB Function/7(setpoint)
  sensorDerivada/1 -> MATLAB Function/9(sensorDerivada)
  Constant1/1 -> MATLAB Function/2(ki)
  Constant3/1 -> MATLAB Function/4(kff)
  Constant4/1 -> MATLAB Function/5(limIntegral)
  Constant5/1 -> MATLAB Function/6(limTotal)
  habIntegral/1 -> MATLAB Function/10(habIntegral)
  Constant2/1 -> MATLAB Function/3(kd)
  Constant/1 -> MATLAB Function/1(kp)

== system Simulador_No_lineal/Sistema de control/PID yaw ==
  setpoint : Inport
  sensor : Inport  Port=2
  sensorDerivada : Inport  Port=3
  habIntegral : Inport  Port=4
  tiempo : Inport  Port=5
  Constant : Constant  Value=Kp
  Constant1 : Constant  Value=Ki
  Constant2 : Constant  Value=Kd
  Constant3 : Constant  Value=Kff
  Constant4 : Constant  Value=LimI
  Constant5 : Constant  Value=LimT
  MATLAB Function : MATLAB Function  TreatAsAtomicUnit=on
  u : Outport
  wires:
  MATLAB Function/1(u) -> u/1
  tiempo/1 -> MATLAB Function/11(tiempo)
  sensor/1 -> MATLAB Function/8(sensor)
  setpoint/1 -> MATLAB Function/7(setPoint)
  sensorDerivada/1 -> MATLAB Function/9(sensorDerivada)
  Constant1/1 -> MATLAB Function/2(ki)
  Constant3/1 -> MATLAB Function/4(kff)
  Constant4/1 -> MATLAB Function/5(limIntegral)
  Constant5/1 -> MATLAB Function/6(limTotal)
  habIntegral/1 -> MATLAB Function/10(habIntegral)
  Constant2/1 -> MATLAB Function/3(kd)
  Constant/1 -> MATLAB Function/1(kp)

== system Simulador_No_lineal/Sistema de control/PID yaw velocidad ==
  setpoint : Inport
  sensor : Inport  Port=2
  sensorDerivada : Inport  Port=3
  habIntegral : Inport  Port=4
  tiempo : Inport  Port=5
  Constant : Constant  Value=Kp
  Constant1 : Constant  Value=Ki
  Constant2 : Constant  Value=Kd
  Constant3 : Constant  Value=Kff
  Constant4 : Constant  Value=LimI
  Constant5 : Constant  Value=LimT
  MATLAB Function : MATLAB Function  TreatAsAtomicUnit=on
  u : Outport
  wires:
  Constant/1 -> MATLAB Function/1(kp)
  Constant2/1 -> MATLAB Function/3(kd)
  habIntegral/1 -> MATLAB Function/10(habIntegral)
  Constant5/1 -> MATLAB Function/6(limTotal)
  Constant4/1 -> MATLAB Function/5(limIntegral)
  Constant3/1 -> MATLAB Function/4(kff)
  Constant1/1 -> MATLAB Function/2(ki)
  sensorDerivada/1 -> MATLAB Function/9(sensorDerivada)
  setpoint/1 -> MATLAB Function/7(setPoint)
  sensor/1 -> MATLAB Function/8(sensor)
  tiempo/1 -> MATLAB Function/11(tiempo)
  MATLAB Function/1(u) -> u/1

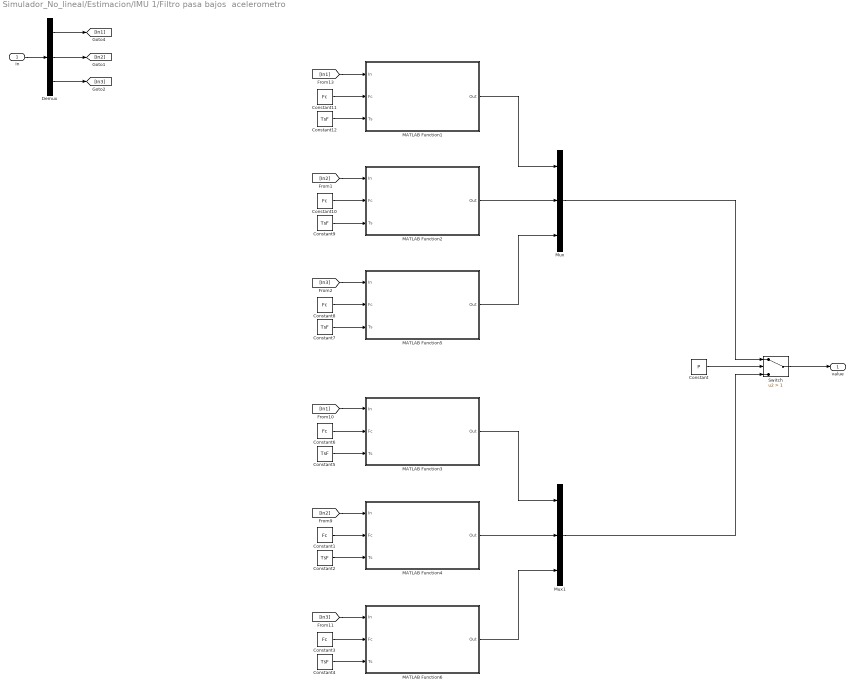
== system Simulador_No_lineal/Estimacion/IMU 1/Filtro pasa bajos  acelerometro ==
  In : Inport
  Constant : Constant  Value=P
  Constant{1,3,6,8,10..11} (6 alike) : Constant  Value=Fc
  Constant{2,4..5,7,9,12} (6 alike) : Constant  Value=TsF
  Demux : Demux  Outputs=3
  MATLAB Function1 : MATLAB Function  TreatAsAtomicUnit=on
  MATLAB Function2 : MATLAB Function  TreatAsAtomicUnit=on
  MATLAB Function3 : MATLAB Function  TreatAsAtomicUnit=on
  MATLAB Function4 : MATLAB Function  TreatAsAtomicUnit=on
  MATLAB Function5 : MATLAB Function  TreatAsAtomicUnit=on
  MATLAB Function6 : MATLAB Function  TreatAsAtomicUnit=on
  Mux : Mux  Inputs=3
  Mux1 : Mux  Inputs=3
  Switch : Switch  Criteria=u2 > Threshold  Threshold=1  SaturateOnIntegerOverflow=off  InputSameDT=off
  value : Outport
  wires:
  Constant/1 -> Switch/2
  Switch/1 -> value/1
  [In1] -> MATLAB Function1/1(In)
  MATLAB Function2/1(Out) -> Mux/2
  MATLAB Function1/1(Out) -> Mux/1
  MATLAB Function5/1(Out) -> Mux/3
  Mux/1 -> Switch/1
  In/1 -> Demux/1
  Demux/1 -> [In1]
  Demux/2 -> [In2]
  Demux/3 -> [In3]
  [In2] -> MATLAB Function2/1(In)
  [In3] -> MATLAB Function5/1(In)
  Constant4/1 -> MATLAB Function6/3(Ts)
  Constant3/1 -> MATLAB Function6/2(Fc)
  Constant1/1 -> MATLAB Function4/2(Fc)
  Constant2/1 -> MATLAB Function4/3(Ts)
  [In3] -> MATLAB Function6/1(In)
  [In2] -> MATLAB Function4/1(In)
  [In1] -> MATLAB Function3/1(In)
  MATLAB Function3/1(Out) -> Mux1/1
  MATLAB Function4/1(Out) -> Mux1/2
  MATLAB Function6/1(Out) -> Mux1/3
  Mux1/1 -> Switch/3
  Constant5/1 -> MATLAB Function3/3(Ts)
  Constant6/1 -> MATLAB Function3/2(Fc)
  Constant7/1 -> MATLAB Function5/3(Ts)
  Constant8/1 -> MATLAB Function5/2(Fc)
  Constant10/1 -> MATLAB Function2/2(Fc)
  Constant9/1 -> MATLAB Function2/3(Ts)
  Constant12/1 -> MATLAB Function1/3(Ts)
  Constant11/1 -> MATLAB Function1/2(Fc)

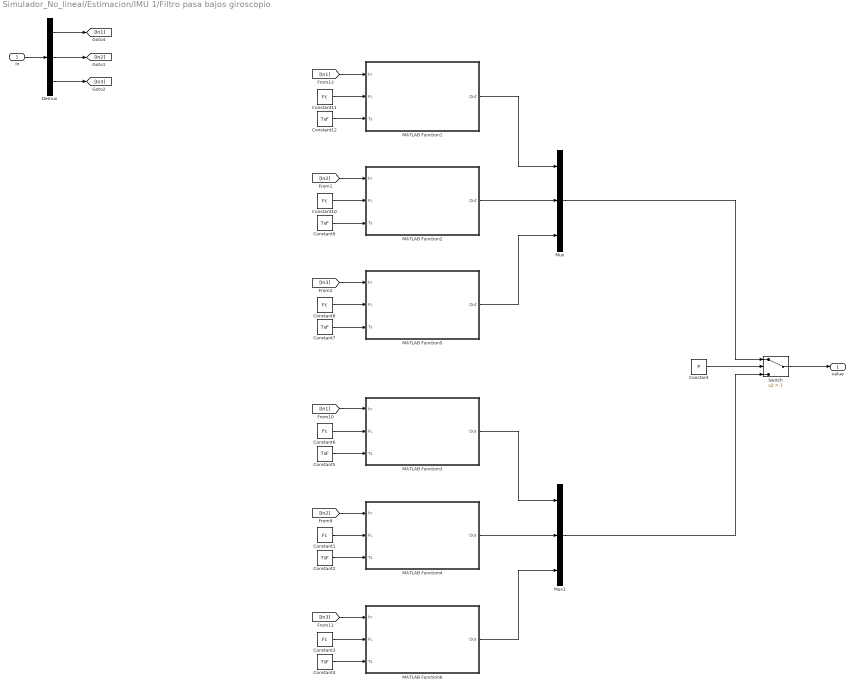
== system Simulador_No_lineal/Estimacion/IMU 1/Filtro pasa bajos giroscopio ==
  In : Inport
  Constant : Constant  Value=P
  Constant{1,3,6,8,10..11} (6 alike) : Constant  Value=Fc
  Constant{2,4..5,7,9,12} (6 alike) : Constant  Value=TsF
  Demux : Demux  Outputs=3
  MATLAB Function1 : MATLAB Function  TreatAsAtomicUnit=on
  MATLAB Function2 : MATLAB Function  TreatAsAtomicUnit=on
  MATLAB Function3 : MATLAB Function  TreatAsAtomicUnit=on
  MATLAB Function4 : MATLAB Function  TreatAsAtomicUnit=on
  MATLAB Function5 : MATLAB Function  TreatAsAtomicUnit=on
  MATLAB Function6 : MATLAB Function  TreatAsAtomicUnit=on
  Mux : Mux  Inputs=3
  Mux1 : Mux  Inputs=3
  Switch : Switch  Criteria=u2 > Threshold  Threshold=1  SaturateOnIntegerOverflow=off  InputSameDT=off
  value : Outport
  wires:
  Constant11/1 -> MATLAB Function1/2(Fc)
  Constant12/1 -> MATLAB Function1/3(Ts)
  Constant9/1 -> MATLAB Function2/3(Ts)
  Constant10/1 -> MATLAB Function2/2(Fc)
  Constant8/1 -> MATLAB Function5/2(Fc)
  Constant7/1 -> MATLAB Function5/3(Ts)
  Constant6/1 -> MATLAB Function3/2(Fc)
  Constant5/1 -> MATLAB Function3/3(Ts)
  Mux1/1 -> Switch/3
  MATLAB Function6/1(Out) -> Mux1/3
  MATLAB Function4/1(Out) -> Mux1/2
  MATLAB Function3/1(Out) -> Mux1/1
  [In1] -> MATLAB Function3/1(In)
  [In2] -> MATLAB Function4/1(In)
  [In3] -> MATLAB Function6/1(In)
  Constant2/1 -> MATLAB Function4/3(Ts)
  Constant1/1 -> MATLAB Function4/2(Fc)
  Constant3/1 -> MATLAB Function6/2(Fc)
  Constant4/1 -> MATLAB Function6/3(Ts)
  [In3] -> MATLAB Function5/1(In)
  [In2] -> MATLAB Function2/1(In)
  Demux/3 -> [In3]
  Demux/2 -> [In2]
  Demux/1 -> [In1]
  In/1 -> Demux/1
  Mux/1 -> Switch/1
  MATLAB Function5/1(Out) -> Mux/3
  MATLAB Function1/1(Out) -> Mux/1
  MATLAB Function2/1(Out) -> Mux/2
  [In1] -> MATLAB Function1/1(In)
  Switch/1 -> value/1
  Constant/1 -> Switch/2

== system Simulador_No_lineal/Estimacion/IMU 1/Sensor IMU ==
  GirT : Inport
  AcelT : Inport  Port=2
  Q : Inport  Port=3
  Constant : Constant  Value=R
  Constant1 : Constant  Value=R
  Gain1 : Gain  Gain=pi/180
  Gain3 : Gain  Gain=180/pi
  Gain4 : Gain  Gain=1/9.81
  IMU : mspsensorlib/IMU  DispRefFrame=NED  Temperature=25  MagneticFieldNED=[ 27.5550, -2.4169, -16.0849 ]  MagneticFieldENU=[ -2.4169, 27.5550, 16.0849 ]  SeedDouble=67  SimulateUsing=Code generation  AccelParamsMeasurementRange=156.9048  AccelParamsResolution=0  AccelParamsConstantBias=[0.0 0.0 0.0]  AccelParamsAxesMisalignment=[0 0 0]  AccelParamsNoiseDensity=aN  AccelParamsBiasInstability=aB  AccelParamsRandomWalk=aK  AccelParamsTemperatureBias=[0 0 0]  AccelParamsTemperatureScaleFactor=[0 0 0]  GyroParamsMeasurementRange=34.9066  GyroParamsResolution=0  GyroParamsConstantBias=[0.0 0.0 0.0]  GyroParamsAxesMisalignment=0  GyroParamsAccelerationBias=[0 0 0]  GyroParamsNoiseDensity=gN  GyroParamsBiasInstability=gB  GyroParamsRandomWalk=gK  GyroParamsTemperatureBias=[0 0 0]  GyroParamsTemperatureScaleFactor=[0 0 0]  MagParamsMeasurementRange=1000  MagParamsResolution=0.1  MagParamsConstantBias=0  MagParamsAxesMisalignment=[0 0 0]  MagParamsNoiseDensity=[0.0424 0.0424 0.0424]  MagParamsBiasInstability=[0 0 0]  MagParamsRandomWalk=[0 0 0]  MagParamsTemperatureBias=[0 0 0]  MagParamsTemperatureScaleFactor=[0 0 0]
  MATLAB Function5 : MATLAB Function  TreatAsAtomicUnit=on  SystemSampleTime=Ts
  Mux : Mux  Inputs=3
  Mux1 : Mux  Inputs=3
  Random Number : RandomNumber  Variance=0.1492^2*1000  SampleTime=Ts
  Random Number3 : RandomNumber  Variance=0.0154^2*1000  SampleTime=Ts
  Sum : Sum  Inputs=|++
  Sum1 : Sum  Inputs=|++
  Switch1 : Switch  Criteria=u2 > Threshold  SaturateOnIntegerOverflow=off  InputSameDT=off
  Switch2 : Switch  Criteria=u2 > Threshold  SaturateOnIntegerOverflow=off  InputSameDT=off
  Transpose1 : Math  Operator=transpose
  Transpose2 : Math  Operator=transpose
  Transpose3 : Math  Operator=transpose
  Zero-Order Hold : ZeroOrderHold  SampleTime=Ts
  Zero-Order Hold1 : ZeroOrderHold  SampleTime=Ts
  Zero-Order Hold2 : ZeroOrderHold  SampleTime=Ts
  AcelB : Outport
  VelB : Outport  Port=2
  wires:
  Gain3/1 -> VelB/1
  Gain4/1 -> AcelB/1
  Transpose1/1 -> Gain4/1
  AcelT/1 -> Zero-Order Hold/1
  GirT/1 -> Zero-Order Hold1/1
  IMU/2 -> Transpose3/1
  IMU/1 -> Transpose1/1
  Transpose3/1 -> Gain3/1
  MATLAB Function5/1(Vel) -> Gain1/1
  Q/1 -> Zero-Order Hold2/1
  Random Number/1 -> Mux/2, Mux/3, Mux/1
  Mux/1 -> Sum/1
  Transpose2/1 -> Switch2/3, Sum/2
  Mux1/1 -> Sum1/1
  Random Number3/1 -> Mux1/1, Mux1/2, Mux1/3
  Sum/1 -> Switch2/1
  Constant/1 -> Switch2/2
  Constant1/1 -> Switch1/2
  Sum1/1 -> Switch1/1
  Gain1/1 -> Switch1/3, Sum1/2
  Switch2/1 -> IMU/1
  Switch1/1 -> IMU/2
  Zero-Order Hold/1 -> Transpose2/1
  Zero-Order Hold1/1 -> MATLAB Function5/1(Wb)
  Zero-Order Hold2/1 -> IMU/3, MATLAB Function5/2(Q)

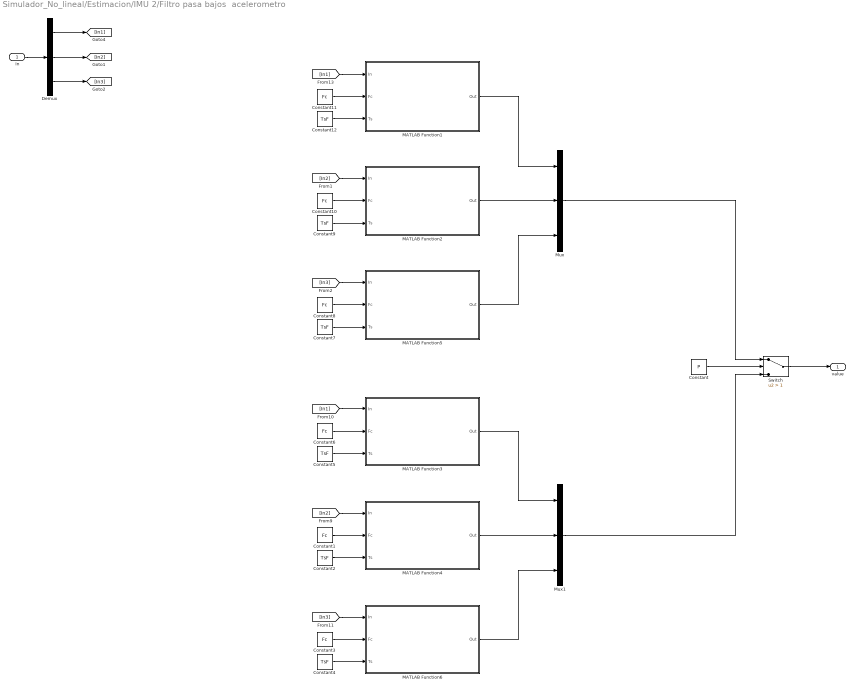
== system Simulador_No_lineal/Estimacion/IMU 2/Filtro pasa bajos  acelerometro ==
  In : Inport
  Constant : Constant  Value=P
  Constant{1,3,6,8,10..11} (6 alike) : Constant  Value=Fc
  Constant{2,4..5,7,9,12} (6 alike) : Constant  Value=TsF
  Demux : Demux  Outputs=3
  MATLAB Function1 : MATLAB Function  TreatAsAtomicUnit=on
  MATLAB Function2 : MATLAB Function  TreatAsAtomicUnit=on
  MATLAB Function3 : MATLAB Function  TreatAsAtomicUnit=on
  MATLAB Function4 : MATLAB Function  TreatAsAtomicUnit=on
  MATLAB Function5 : MATLAB Function  TreatAsAtomicUnit=on
  MATLAB Function6 : MATLAB Function  TreatAsAtomicUnit=on
  Mux : Mux  Inputs=3
  Mux1 : Mux  Inputs=3
  Switch : Switch  Criteria=u2 > Threshold  Threshold=1  SaturateOnIntegerOverflow=off  InputSameDT=off
  value : Outport
  wires:
  Constant11/1 -> MATLAB Function1/2(Fc)
  Constant12/1 -> MATLAB Function1/3(Ts)
  Constant9/1 -> MATLAB Function2/3(Ts)
  Constant10/1 -> MATLAB Function2/2(Fc)
  Constant8/1 -> MATLAB Function5/2(Fc)
  Constant7/1 -> MATLAB Function5/3(Ts)
  Constant6/1 -> MATLAB Function3/2(Fc)
  Constant5/1 -> MATLAB Function3/3(Ts)
  Mux1/1 -> Switch/3
  MATLAB Function6/1(Out) -> Mux1/3
  MATLAB Function4/1(Out) -> Mux1/2
  MATLAB Function3/1(Out) -> Mux1/1
  [In1] -> MATLAB Function3/1(In)
  [In2] -> MATLAB Function4/1(In)
  [In3] -> MATLAB Function6/1(In)
  Constant2/1 -> MATLAB Function4/3(Ts)
  Constant1/1 -> MATLAB Function4/2(Fc)
  Constant3/1 -> MATLAB Function6/2(Fc)
  Constant4/1 -> MATLAB Function6/3(Ts)
  [In3] -> MATLAB Function5/1(In)
  [In2] -> MATLAB Function2/1(In)
  Demux/3 -> [In3]
  Demux/2 -> [In2]
  Demux/1 -> [In1]
  In/1 -> Demux/1
  Mux/1 -> Switch/1
  MATLAB Function5/1(Out) -> Mux/3
  MATLAB Function1/1(Out) -> Mux/1
  MATLAB Function2/1(Out) -> Mux/2
  [In1] -> MATLAB Function1/1(In)
  Switch/1 -> value/1
  Constant/1 -> Switch/2

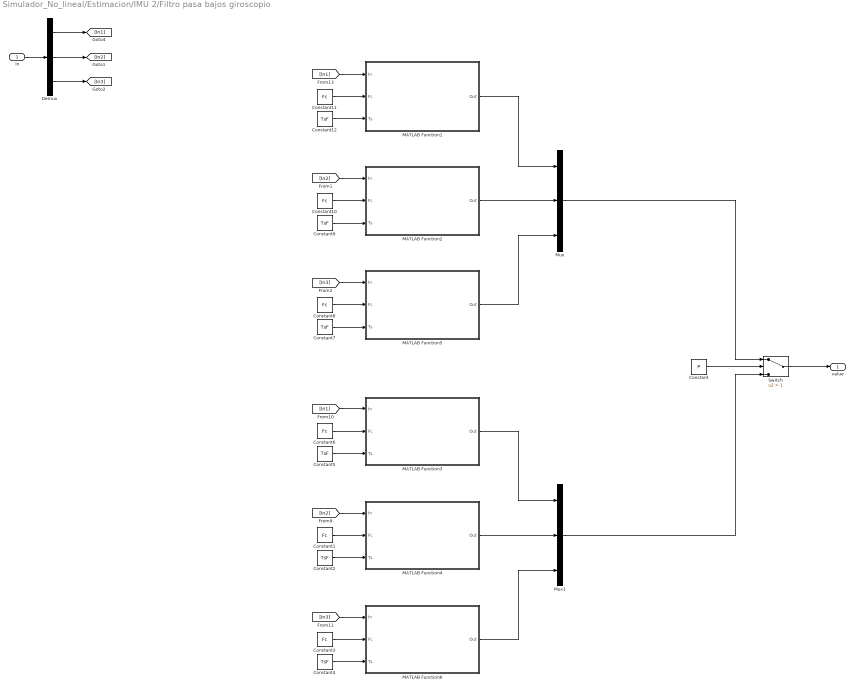
== system Simulador_No_lineal/Estimacion/IMU 2/Filtro pasa bajos giroscopio ==
  In : Inport
  Constant : Constant  Value=P
  Constant{1,3,6,8,10..11} (6 alike) : Constant  Value=Fc
  Constant{2,4..5,7,9,12} (6 alike) : Constant  Value=TsF
  Demux : Demux  Outputs=3
  MATLAB Function1 : MATLAB Function  TreatAsAtomicUnit=on
  MATLAB Function2 : MATLAB Function  TreatAsAtomicUnit=on
  MATLAB Function3 : MATLAB Function  TreatAsAtomicUnit=on
  MATLAB Function4 : MATLAB Function  TreatAsAtomicUnit=on
  MATLAB Function5 : MATLAB Function  TreatAsAtomicUnit=on
  MATLAB Function6 : MATLAB Function  TreatAsAtomicUnit=on
  Mux : Mux  Inputs=3
  Mux1 : Mux  Inputs=3
  Switch : Switch  Criteria=u2 > Threshold  Threshold=1  SaturateOnIntegerOverflow=off  InputSameDT=off
  value : Outport
  wires:
  Constant/1 -> Switch/2
  Switch/1 -> value/1
  [In1] -> MATLAB Function1/1(In)
  MATLAB Function2/1(Out) -> Mux/2
  MATLAB Function1/1(Out) -> Mux/1
  MATLAB Function5/1(Out) -> Mux/3
  Mux/1 -> Switch/1
  In/1 -> Demux/1
  Demux/1 -> [In1]
  Demux/2 -> [In2]
  Demux/3 -> [In3]
  [In2] -> MATLAB Function2/1(In)
  [In3] -> MATLAB Function5/1(In)
  Constant4/1 -> MATLAB Function6/3(Ts)
  Constant3/1 -> MATLAB Function6/2(Fc)
  Constant1/1 -> MATLAB Function4/2(Fc)
  Constant2/1 -> MATLAB Function4/3(Ts)
  [In3] -> MATLAB Function6/1(In)
  [In2] -> MATLAB Function4/1(In)
  [In1] -> MATLAB Function3/1(In)
  MATLAB Function3/1(Out) -> Mux1/1
  MATLAB Function4/1(Out) -> Mux1/2
  MATLAB Function6/1(Out) -> Mux1/3
  Mux1/1 -> Switch/3
  Constant5/1 -> MATLAB Function3/3(Ts)
  Constant6/1 -> MATLAB Function3/2(Fc)
  Constant7/1 -> MATLAB Function5/3(Ts)
  Constant8/1 -> MATLAB Function5/2(Fc)
  Constant10/1 -> MATLAB Function2/2(Fc)
  Constant9/1 -> MATLAB Function2/3(Ts)
  Constant12/1 -> MATLAB Function1/3(Ts)
  Constant11/1 -> MATLAB Function1/2(Fc)
